simulink model "model"  (R2020a)
settings: Solver=VariableStepAuto  StartTime=0.0  StopTime=10  RelTol=1e-3
settings Model: Creator=VicenteRivera  LastModifiedBy=VicenteRivera

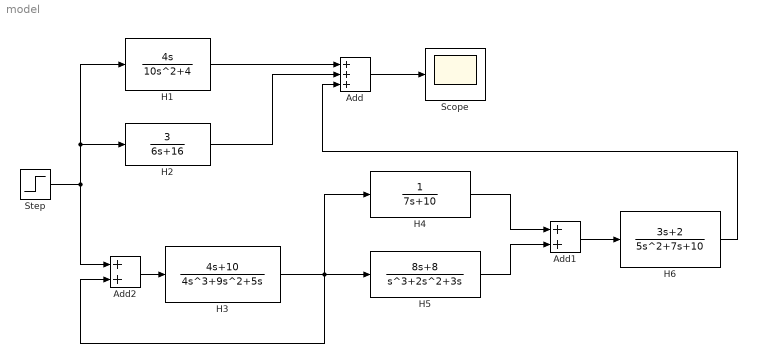
== system model ==
  Add : Sum  Inputs=+++
  Add1 : Sum
  Add2 : Sum
  H1 : TransferFcn  Numerator=[0 4 0]  Denominator=[10 0 4]  ContinuousStateAttributes='H1'
  H2 : TransferFcn  Numerator=[0 3]  Denominator=[6 16]  ContinuousStateAttributes='H2'
  H3 : TransferFcn  Numerator=[0 4 10]  Denominator=[4 9 5 0]  ContinuousStateAttributes='H3'
  H4 : TransferFcn  Numerator=[0 1]  Denominator=[7 10]  ContinuousStateAttributes='H4'
  H5 : TransferFcn  Numerator=[0 0 8 8]  Denominator=[1 2 3 0]  ContinuousStateAttributes='H5'
  H6 : TransferFcn  Numerator=[0 3 2]  Denominator=[5 7 10]  ContinuousStateAttributes='H6'
  Scope : Scope
  Step : Step  SampleTime=0
  wires:
  H4/1 -> Add1/1
  H5/1 -> Add1/2
  Add1/1 -> H6/1
  Add/1 -> Scope/1
  Add2/1 -> H3/1
  H3/1 -> Add2/2, H4/1, H5/1
  Step/1 -> H1/1, H2/1, Add2/1
  H1/1 -> Add/1
  H2/1 -> Add/2
  H6/1 -> Add/3
